simulink model "cross_multiplier_blk"  (R2019a)
settings: Solver=VariableStepAuto  StartTime=0.0  StopTime=10.0  RelTol=1e-3
libraries: xbsIndex_r4 x1
settings Model: Creator=mybur  LastModifiedBy=mybur

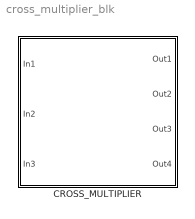
== system cross_multiplier_blk ==
  CROSS_MULTIPLIER : Subsystem  mask{nof_streams=2, aggregation=1, in_bit_w=4, out_bit_w=9, use_gauss=off, use_dsp=on, pipeline_input=1, pipeline_product=1, pipeline_adder=1, pipeline_round=1, pipeline_output=0, ovflw_behav=off, quant_behav=0}
      mask prompts: nof_streams "Number input streams"; aggregation "Aggregation per stream"; in_bit_w "Bit width in"; out_bit_w "Bit width out"; use_gauss "Use Gaussian Cmult?"; use_dsp "Use DSP48 for Cmult?"; pipeline_input "Input latency"; pipeline_product "Product latency"; pipeline_adder "Adder latency"; pipeline_round "Rounding latency"; pipeline_output "Output latency"; ovflw_behav "Saturate overflow"; quant_behav "FFT rounding mode: 0-Truncate, 1-Round Even, 2-Round Infinite"
      mask TypeOptions quant_behav: 0 | 1 | 2

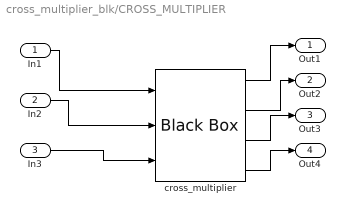
== system cross_multiplier_blk/CROSS_MULTIPLIER ==
  In1 : Inport
  In2 : Inport  Port=2
  In3 : Inport  Port=3
  cross_multiplier : xbsIndex_r4/Black Box  init_code=cross_mult_config  sim_method=ISE Simulator  verbose=off  block_type=blackbox2
  Out1 : Outport
  Out2 : Outport  Port=2
  Out3 : Outport  Port=3
  Out4 : Outport  Port=4
  wires:
  In2/1 -> cross_multiplier/2
  cross_multiplier/4 -> Out4/1
  In1/1 -> cross_multiplier/1
  cross_multiplier/2 -> Out2/1
  cross_multiplier/1 -> Out1/1
  In3/1 -> cross_multiplier/3
  cross_multiplier/3 -> Out3/1
